simulink model "Cycloconverter_with_R_Load"  (R2023b)
settings: Solver=VariableStepAuto  StartTime=0.0  StopTime=0.1  RelTol=1e-3
libraries: spsDetailedThyristorLib x24, spsACVoltageSourceLib x6, spsVoltageMeasurementLib x6, spsCurrentMeasurementLib x3, spsSeriesRLCBranchLib x3, sps_lib x1
settings Model: Creator=HP  LastModifiedBy=HP

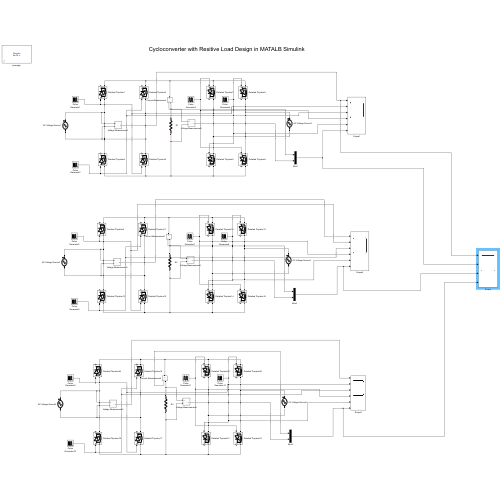
[thumbnail: Simulink's stored preview of the top-level diagram]
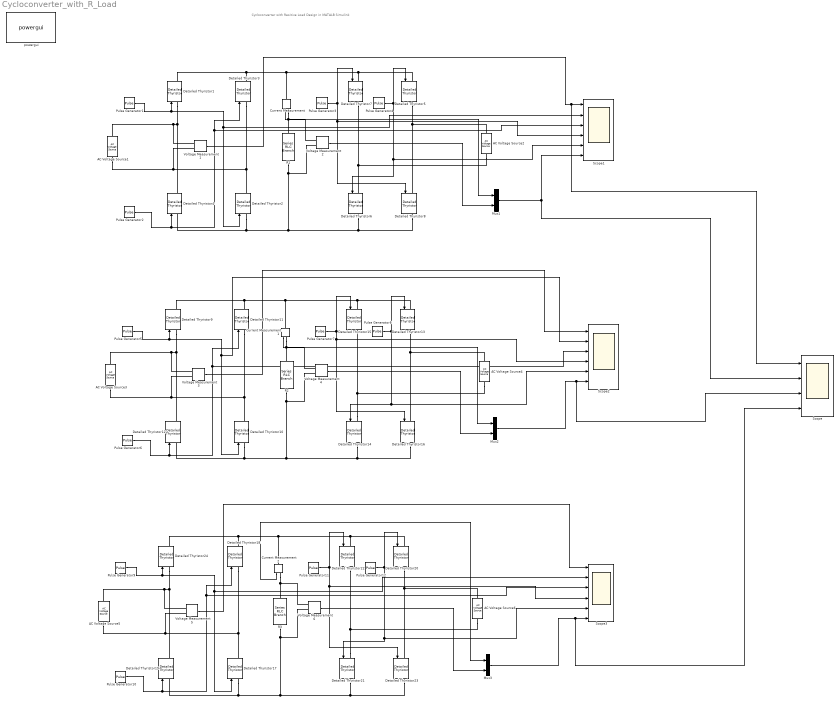
== system Cycloconverter_with_R_Load ==
  note: Cycloconverter with Resitive Load Design in MATALB Simulink
  AC Voltage Source{1..6} (6 alike) : spsACVoltageSourceLib/AC Voltage Source  Amplitude=230  Phase=0  Frequency=50  SampleTime=0  Measurements=None  BusType=swing  Pref=10e3  Qref=0  Qmin=-inf  Qmax=+inf
  Current Measurement : spsCurrentMeasurementLib/Current Measurement  PhasorSimulation=off  OutputType=Complex  PSBequivalent=0
  Current Measurement1 : spsCurrentMeasurementLib/Current Measurement  PhasorSimulation=off  OutputType=Complex  PSBequivalent=0
  Current Measurement2 : spsCurrentMeasurementLib/Current Measurement  PhasorSimulation=off  OutputType=Complex  PSBequivalent=0
  Detailed Thyristor{1..24} (24 alike) : spsDetailedThyristorLib/Detailed Thyristor  Ron=0.001  Lon=1e-3  Vf=0.8  IL=0.1  Tq=100e-6  IC=0  Rs=500  Cs=250e-9  Measurements=on
      settings: LibrarySourceBlock=sps_lib/Power Electronics/Detailed Thyristor
  Mux1 : Mux  Inputs=2
  Mux2 : Mux  Inputs=2
  Mux3 : Mux  Inputs=2
  Pulse Generator1 : DiscretePulseGenerator  PulseType=Time based  Period=0.04  PulseWidth=2  PhaseDelay=0.04*(30)/720
  Pulse Generator10 : DiscretePulseGenerator  PulseType=Time based  Period=0.04  PulseWidth=2  PhaseDelay=0.04*(90+180)/720
  Pulse Generator11 : DiscretePulseGenerator  PulseType=Time based  Period=0.04  PulseWidth=2  PhaseDelay=0.04*(90+180+180)/720
  Pulse Generator12 : DiscretePulseGenerator  PulseType=Time based  Period=0.04  PulseWidth=2  PhaseDelay=0.04*(90+180+180+180)/720
  Pulse Generator2 : DiscretePulseGenerator  PulseType=Time based  Period=0.04  PulseWidth=2  PhaseDelay=0.04*(30+180)/720
  Pulse Generator3 : DiscretePulseGenerator  PulseType=Time based  Period=0.04  PulseWidth=2  PhaseDelay=0.04*(30+180+180)/720
  Pulse Generator4 : DiscretePulseGenerator  PulseType=Time based  Period=0.04  PulseWidth=2  PhaseDelay=0.04*(30+180+180+180)/720
  Pulse Generator5 : DiscretePulseGenerator  PulseType=Time based  Period=0.04  PulseWidth=2  PhaseDelay=0.04*(60)/720
  Pulse Generator6 : DiscretePulseGenerator  PulseType=Time based  Period=0.04  PulseWidth=2  PhaseDelay=0.04*(60+180)/720
  Pulse Generator7 : DiscretePulseGenerator  PulseType=Time based  Period=0.04  PulseWidth=2  PhaseDelay=0.04*(60+180+180)/720
  Pulse Generator8 : DiscretePulseGenerator  PulseType=Time based  Period=0.04  PulseWidth=2  PhaseDelay=0.04*(60+180+180+180)/720
  Pulse Generator9 : DiscretePulseGenerator  PulseType=Time based  Period=0.04  PulseWidth=2  PhaseDelay=0.04*(90)/720
  R1 : spsSeriesRLCBranchLib/Series RLC Branch  LConnTagsString=__new0  RConnTagsString=__new0  BranchType=R  Resistance=2  Inductance=1e-3  SetiL0=off  InitialCurrent=0  Capacitance=1e-6  Setx0=off  InitialVoltage=0  Measurements=None
  R2 : spsSeriesRLCBranchLib/Series RLC Branch  LConnTagsString=__new0  RConnTagsString=__new0  BranchType=R  Resistance=2  Inductance=1e-3  SetiL0=off  InitialCurrent=0  Capacitance=1e-6  Setx0=off  InitialVoltage=0  Measurements=None
  R3 : spsSeriesRLCBranchLib/Series RLC Branch  LConnTagsString=__new0  RConnTagsString=__new0  BranchType=R  Resistance=2  Inductance=1e-3  SetiL0=off  InitialCurrent=0  Capacitance=1e-6  Setx0=off  InitialVoltage=0  Measurements=None
  Scope : Scope  NumInputPorts=4
  Scope1 : Scope  NumInputPorts=6
  Scope2 : Scope  NumInputPorts=6
  Scope3 : Scope  NumInputPorts=6
  Voltage Measurement{1..6} (6 alike) : spsVoltageMeasurementLib/Voltage Measurement  PhasorSimulation=off  OutputType=Complex  PSBequivalent=0
  powergui : sps_lib/powergui  Priority=1  SimulationMode=Discrete  SampleTime=50e-6  frequency=60  Iterations=50  frequencyindice=50  Pbase=100e6  ErrMax=1e-4  UnitsV=kV  UnitsW=MW  buscounter=0  FunctionMessages=off  echomessages=off  EnableUseOfTLC=off  CurrentSourceSwitches=off  DisableSnubberDevices=off  DisableRonSwitches=off  DisableVfSwitches=off  DisplayEquations=off  AutomaticDiscreteSolvers=off  SolverType=Tustin/Backward Euler (TBE)  Interpol=off  ExternalGateDelay=off  methode=off  Ts=100  x0status=blocks  SPID=on  SwTol=0  HookPort=off  NonlinearTolerance=1e-4  nMaxIteration=100  ContinueOnMaxIteration=off  RestoreLinks=warning  ResistiveCurrentMeasurement=off  Frange=[0:2:500]  Ylog=off  Xlog=on  ShowGrid=off  save=off  variable=ZData  structure=0  ZoomFFT=off  StartTime=0.0  cycles=1  DisplayStyle=1  fundamental=60  FreqAxis=off  MaxFrequency=1000  frequencyindicesteady=1  RmsSteady=1  display=off
  wires:
  Pulse Generator1/1 -> Scope1/2, Detailed Thyristor2/1, Detailed Thyristor1/1
  Pulse Generator2/1 -> Detailed Thyristor3/1, Scope1/3, Detailed Thyristor4/1
  Pulse Generator3/1 -> Detailed Thyristor8/1, Scope1/4, Detailed Thyristor7/1
  Pulse Generator4/1 -> Detailed Thyristor6/1, Scope1/5, Detailed Thyristor5/1
  Voltage Measurement1/1 -> Scope1/1, Scope/1
  Current Measurement/1 -> Mux1/1
  Voltage Measurement2/1 -> Mux1/2
  Mux1/1 -> Scope/2, Scope1/6
  Pulse Generator8/1 -> Detailed Thyristor14/1, Scope2/5, Detailed Thyristor13/1
  Mux2/1 -> Scope2/6, Scope/3
  Pulse Generator7/1 -> Detailed Thyristor16/1, Scope2/4, Detailed Thyristor15/1
  Pulse Generator6/1 -> Detailed Thyristor11/1, Scope2/3, Detailed Thyristor12/1
  Voltage Measurement4/1 -> Mux2/2
  Voltage Measurement3/1 -> Scope2/1
  Current Measurement1/1 -> Mux2/1
  Pulse Generator5/1 -> Scope2/2, Detailed Thyristor10/1, Detailed Thyristor9/1
  Current Measurement2/1 -> Mux3/1
  Pulse Generator11/1 -> Detailed Thyristor23/1, Scope3/4, Detailed Thyristor22/1
  Voltage Measurement6/1 -> Mux3/2
  Pulse Generator10/1 -> Scope3/3, Detailed Thyristor18/1, Detailed Thyristor19/1
  Pulse Generator9/1 -> Scope3/2, Detailed Thyristor17/1, Detailed Thyristor24/1
  Pulse Generator12/1 -> Detailed Thyristor21/1, Scope3/5, Detailed Thyristor20/1
  Voltage Measurement5/1 -> Scope3/1
  Mux3/1 -> Scope3/6, Scope/4
  connections:
  Detailed Thyristor1/LConn1 -- Voltage Measurement1/LConn1 -- AC Voltage Source1/RConn1 -- Detailed Thyristor4/RConn1
  Detailed Thyristor3/LConn1 -- Voltage Measurement1/LConn2 -- AC Voltage Source1/LConn1 -- Detailed Thyristor2/RConn1
  Detailed Thyristor7/RConn1 -- AC Voltage Source2/LConn1 -- Detailed Thyristor6/LConn1
  Detailed Thyristor5/RConn1 -- Detailed Thyristor8/LConn1 -- AC Voltage Source2/RConn1
  Detailed Thyristor3/RConn1 -- Detailed Thyristor5/LConn1 -- Detailed Thyristor7/LConn1 -- Current Measurement/LConn1 -- Detailed Thyristor1/RConn1
  Detailed Thyristor2/LConn1 -- R1/LConn1 -- Voltage Measurement2/LConn2 -- Detailed Thyristor6/RConn1 -- Detailed Thyristor8/RConn1 -- Detailed Thyristor4/LConn1
  Voltage Measurement2/LConn1 -- Current Measurement/RConn1 -- R1/RConn1
  Detailed Thyristor12/LConn1 -- Detailed Thyristor10/LConn1 -- R2/LConn1 -- Voltage Measurement4/LConn2 -- Detailed Thyristor14/RConn1 -- Detailed Thyristor16/RConn1
  Voltage Measurement4/LConn1 -- Current Measurement1/RConn1 -- R2/RConn1
  AC Voltage Source3/RConn1 -- Voltage Measurement3/LConn1 -- Detailed Thyristor12/RConn1 -- Detailed Thyristor9/LConn1
  Detailed Thyristor15/LConn1 -- Detailed Thyristor13/LConn1 -- Current Measurement1/LConn1 -- Detailed Thyristor11/RConn1 -- Detailed Thyristor9/RConn1
  Detailed Thyristor14/LConn1 -- Detailed Thyristor15/RConn1 -- AC Voltage Source4/LConn1
  Detailed Thyristor13/RConn1 -- Detailed Thyristor16/LConn1 -- AC Voltage Source4/RConn1
  Detailed Thyristor11/LConn1 -- Voltage Measurement3/LConn2 -- AC Voltage Source3/LConn1 -- Detailed Thyristor10/RConn1
  Detailed Thyristor18/LConn1 -- Voltage Measurement5/LConn2 -- AC Voltage Source5/LConn1 -- Detailed Thyristor17/RConn1
  AC Voltage Source5/RConn1 -- Voltage Measurement5/LConn1 -- Detailed Thyristor19/RConn1 -- Detailed Thyristor24/LConn1
  Detailed Thyristor22/LConn1 -- Detailed Thyristor20/LConn1 -- Current Measurement2/LConn1 -- Detailed Thyristor18/RConn1 -- Detailed Thyristor24/RConn1
  Detailed Thyristor20/RConn1 -- Detailed Thyristor23/LConn1 -- AC Voltage Source6/RConn1
  Detailed Thyristor21/LConn1 -- Detailed Thyristor22/RConn1 -- AC Voltage Source6/LConn1
  Voltage Measurement6/LConn1 -- Current Measurement2/RConn1 -- R3/RConn1
  Detailed Thyristor19/LConn1 -- Detailed Thyristor17/LConn1 -- R3/LConn1 -- Voltage Measurement6/LConn2 -- Detailed Thyristor21/RConn1 -- Detailed Thyristor23/RConn1
